simulink model "SF053A_HwAgVehCentrTrim"  (R2013b)
settings: Solver=FixedStepDiscrete  SolverMode=SingleTasking  StartTime=0.0  StopTime=1  FixedStep=0.002  RelTol=1e-3
values from neighbouring files (symbols this model uses):
  ENGRUNACTVTRUE_CNT_U08 = DataDict.Constant    [SF053A_HwAgVehCentrTrim_DataDict.m]
  HWAGCLRTRIMPRFMD_CNT_LGC = DataDict.Constant    [SF053A_HwAgVehCentrTrim_DataDict.m]
  HWAGCLRVAL_HWDEG_F32 = DataDict.Constant    [SF053A_HwAgVehCentrTrim_DataDict.m]
  HWAGEOTCCWNOTDETD_CNT_U08 = DataDict.Constant    [SF053A_HwAgVehCentrTrim_DataDict.m]
  HWAGEOTCWNOTDETD_CNT_U08 = DataDict.Constant    [SF053A_HwAgVehCentrTrim_DataDict.m]
  HWAGMAGTHDEXCDD_CNT_U08 = DataDict.Constant    [SF053A_HwAgVehCentrTrim_DataDict.m]
  HWAGTRIMPRFMD_CNT_LGC = DataDict.Constant    [SF053A_HwAgVehCentrTrim_DataDict.m]
  HwAgVehCentrTrimHwAgLim = DataDict.Calibration    [SF053A_HwAgVehCentrTrim_DataDict.m]
  HwAgVehCentrTrimVehSpdMaxThd = DataDict.Calibration    [SF053A_HwAgVehCentrTrim_DataDict.m]
  HwAgVehCentrTrimVld = DataDict.NTC    [SF053A_HwAgVehCentrTrim_DataDict.m]
  NODEBSTEP_CNT_U16 = DataDict.Constant    [SF053A_HwAgVehCentrTrim_DataDict.m]
  UPDHWAGTRIMPRFMD_CNT_U08 = DataDict.Constant    [SF053A_HwAgVehCentrTrim_DataDict.m]
  VEHSPDTHDEXCDD_CNT_U08 = DataDict.Constant    [SF053A_HwAgVehCentrTrim_DataDict.m]
undefined symbols (not defined in the file or in its folder): NtcSts1, u2, u3, u4, u5
libraries: simulink x6, NxtrNvM x3, NxtrLim x2
(part 1 of 3)
settings Model: Creator=qzwc4r  LastModifiedBy=NZ2883
settings SolverCC: AutoInsertRateTranBlk=on  InsertRTBMode=Always
settings DataIOCC: LimitDataPoints=off  SaveFormat=Structure  ReturnWorkspaceOutputs=on
settings OptimizationCC: BlockReduction=off  InlineParams=on  ZeroExternalMemoryAtStartup=off  ZeroInternalMemoryAtStartup=off  OptimizeModelRefInitCode=on  LifeSpan=1
settings DebuggingCC: SignalInfNanChecking=error  SignalRangeChecking=warning  UnderspecifiedInitializationDetection=Simplified  SolverPrmCheckMsg=error  InheritedTsInSrcMsg=error  DiscreteInheritContinuousMsg=error  SingleTaskRateTransMsg=error  TasksWithSamePriorityMsg=error  SigSpecEnsureSampleTimeMsg=error  CheckMatrixSingularityMsg=error  ParameterUnderflowMsg=error  ParameterPrecisionLossMsg=error  ParameterTunabilityLossMsg=error  FixptConstUnderflowMsg=warning  FixptConstOverflowMsg=warning  VectorMatrixConversionMsg=error  SignalLabelMismatchMsg=error  UnconnectedInputMsg=error  UnconnectedOutputMsg=error  UnconnectedLineMsg=error  SFcnCompatibilityMsg=error  UniqueDataStoreMsg=warning  BusObjectLabelMismatch=error  RootOutportRequireBusObject=error  AssertControl=DisableAll  ModelReferenceIOMsg=error  ModelReferenceVersionMismatchMessage=warning  ModelReferenceIOMismatchMessage=error  ModelReferenceCSMismatchMessage=warning  ModelReferenceDataLoggingMessage=error  StateNameClashWarn=warning  StrictBusMsg=ErrorOnBusTreatedAsVector  NonBusSignalsTreatedAsBus=error  SFUnexpectedBacktrackingDiag=error  SFInvalidInputDataAccessInChartInitDiag=error  SFNoUnconditionalDefaultTransitionDiag=error  SFTransitionOutsideNaturalParentDiag=error  SFUnconditionalTransitionShadowingDiag=error  SFUndirectedBroadcastEventsDiag=error
settings ModelReferenceCC: ModelReferenceNumInstancesAllowed=Single
settings RTWCC: SystemTargetFile=autosar.tlc  GenCodeOnly=on  TemplateMakefile=ert_default_tmf  Description=AUTOSAR  GenerateReport=on  ProcessScript=autosar_make_rtw_hook  LaunchReport=on
settings CodeAppCC: GenerateComments=off  IgnoreCustomStorageClasses=off  CustomSymbolStrType=$N$R$M  CustomSymbolStrBlkIO=$N$M  SimulinkBlockComments=off
settings STFCustomTargetCC: ParMdlRefBuildCompliant=on  CompOptLevelCompliant=on  IncludeMdlTerminateFcn=off  CombineOutputUpdateFcns=on  SuppressErrorStatus=on  ERTFirstTimeCompliant=on  ERTCustomFileBanners=on  SupportNonFinite=off  SupportComplex=off  SupportContinuousTime=off  SupportNonInlinedSFcns=off  MATLABClassNameForMDSCustomization=Simulink.SoftwareTarget.ERTCustomization  AutosarCompliant=on  GRTInterface=off  SystemTargetFile=autosar.tlc
settings ERTTargetCC: CodeReplacementLibrary=ANSI_C  ConcurrentExecutionCompliant=off  IncludeMdlTerminateFcn=off  SuppressErrorStatus=on  SupportNonFinite=off  SupportComplex=off  ModelStepFunctionPrototypeControlCompliant=off  CPPClassGenCompliant=off  AutosarCompliant=on  InlinedParameterPlacement=NonHierarchical  ERTCustomFileTemplate=example_file_process.tlc  EnableUserReplacementTypes=on

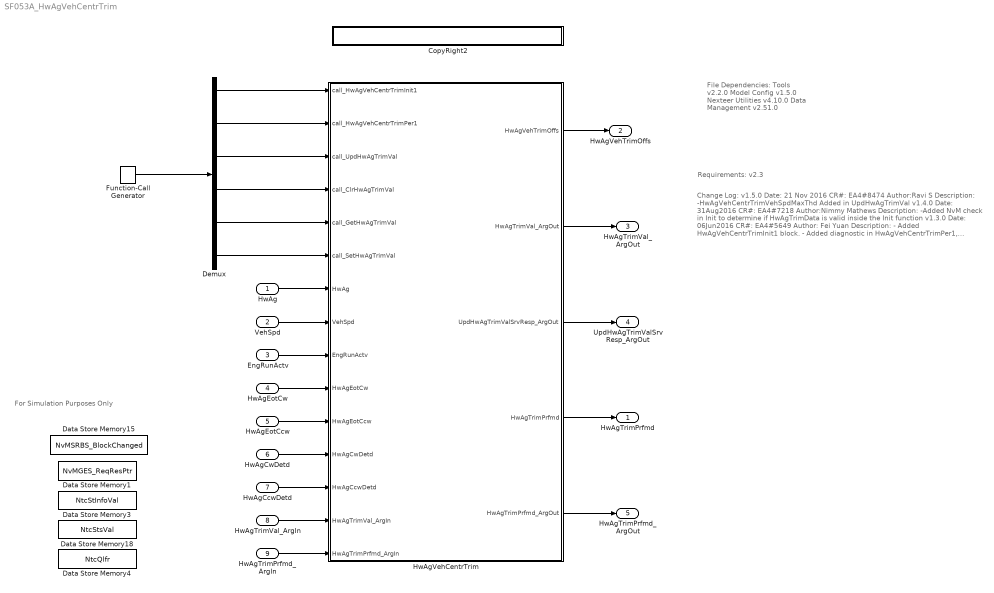
== system SF053A_HwAgVehCentrTrim ==
  note: Requirements: v2.3
  note: File Dependencies:
      | Tools v2.2.0
      | Model Config v1.5.0
      | Nexteer Utilities v4.10.0
      | Data Management v2.51.0
  note: Change Log:
      |
      | v1.5.0
      | Date: 21 Nov 2016
      | CR#: EA4#8474
      | Author:Ravi S
      | Description:
      | -HwAgVehCentrTrimVehSpdMaxThd  Added in UpdHwAgTrimVal
      |
      |
      | v1.4.0
      | Date: 31Aug2016
      | CR#: EA4#7218
      | Author:Nimmy Mathews
      | Description:
      | -Added NvM check in Init to determine if HwAgTrimData is valid inside
      | the Init function
      |
      | v1.3.0
      | Date: 06Jun2016
      | CR#: EA4#5649
      | Author: Fei Yuan
      | Description:
      | - Added HwAgVehCentrTrimInit1 block.
      | - Added diagnostic in HwAgVehCentrTrimPer1,
      |   UpdHwAgTrimVal and ClrHwAgTrimVal.
      | - Added NODEBSTEP_CNT_U16, HwAgVehCentrTrimVld
      |   HWAGVEHCENTRTRIM_HWAGVEHCENTRTRIMVLDNTCNR_CNT_ENUM.
      | - Changed the range of UpdHwAgTrimValSrvResp_ArgOut to [0,5]
      |
      | v1.2.0
      | Date: 4April2016
      | CR#: EA4#4776
      | Author: Nimmy Mathews
      | Description:
      |  - Added default value to the NVM Data Definition
      | in DD
      |
      | v1.1.0
      | Date: 30March2016
      | CR#: EA4#4776
      | Author: Nimmy Mathews
      | Description:
      |  -Added new HwAgTrimPrfmd global output and
      |  also the Trim Performed status written to NVRAM.
      | Two interface names changed
      | -HwAgEotCwDetd is renamed to HwAgCwDetd
      | -HwAgEotCcwDetd is renamed to HwAgCcwDetd
      |
      | v1.0.0
      | Date: 16Feb2016
      | CR#: EA4#3817
      | Author: Price Lefler
      | Description:
      |  - Initial Design
  note: For Simulation Purposes Only
  HwAg : Inport  RequirementInfo={} %GIDa_113f3a3e_16c4_454d_8e42_dd983b59641f
  VehSpd : Inport  RequirementInfo={} %GIDa_04c22129_0294_4664_9901_89f5670e71dd  Port=2
  EngRunActv : Inport  RequirementInfo={} %GIDa_2ca8b555_30d5_45c5_8570_785fbe8b196c  Port=3
  HwAgEotCw : Inport  RequirementInfo={} %GIDa_4439beba_6576_476c_b9c0_099ead0766d6  Port=4
  HwAgEotCcw : Inport  RequirementInfo={} %GIDa_f3262bf3_e9f3_4a2e_972e_ca5eb7281d34  Port=5
  HwAgCwDetd : Inport  RequirementInfo={} %GIDa_8f1cc708_64b7_49e1_8286_e1db8b0c7567  Port=6
  HwAgCcwDetd : Inport  RequirementInfo={} %GIDa_978389ba_efca_48a6_b124_a6774b318c9c  Port=7
  HwAgTrimVal_ArgIn : Inport  RequirementInfo={} %GIDa_c15efb6b_9d38_4c87_8d86_863040277de8  Port=8
  HwAgTrimPrfmd_ArgIn : Inport  RequirementInfo={} %GIDa_654e7d29_ce2a_48b7_b803_7a5262d5d910  Port=9
  CopyRight2 : Subsystem  Description=|  mask(Copyright Information){none=on}
      | Copyright info block.                                               
      |                                                                     
      | Place copyright information at the top of every subsystem in design.
      mask prompts: none "No parameters"
      mask help: Place copyright information at the top of every subsystem in design.
      mask Display:
      | NxtrConf = 'Nexteer Confidential';
      | 
      | sys = bdroot; %handle for the current model ("system")
      | first = get_param(sys,'Created');
      | if(isempty(first))
      |     first = datestr(now,'yyyy');
      | else
      |     first = first(end-3:end);  %year is last four digits
      | end
      | 
      | last = get_param(sys,'LastModifiedDate');
      | if isempty(last)
      |     last = datestr(now,'yyyy');
      | else
      |     last = last(end-3:end);
      | end
      | 
      | if strcmp(first,last)
      |     fprintf('%s -- Copyright %s Nexteer',NxtrConf,first)
      | else
      |     fprintf('%s -- %s%s- %s Nexteer',NxtrConf,char(169),first,last)
      | end
  Data Store Memory1 : DataStoreMemory  DataStoreName=NvMGES_ReqResPtr  OutDataTypeStr=uint8
  Data Store Memory15 : DataStoreMemory  DataStoreName=NvMSRBS_BlockChanged  VectorParams1D=off
  Data Store Memory18 : DataStoreMemory  DataStoreName=NtcStsVal  InitialValue=NtcSts1.NTCSTS_PASSD  OutDataTypeStr=Enum: NtcSts1
  Data Store Memory3 : DataStoreMemory  DataStoreName=NtcStInfoVal  OutDataTypeStr=uint8
  Data Store Memory4 : DataStoreMemory  DataStoreName=NtcQlfr  InitialValue=SigQlfr1.SIGQLFR_NORES  OutDataTypeStr=Enum: SigQlfr1
  Demux : Demux  Outputs=6
  Function-Call Generator : simulink/Ports & Subsystems/Function-Call Generator  sample_time=1  numberOfIterations=1
  HwAgVehCentrTrim : Subsystem
  HwAgTrimPrfmd : Outport
  HwAgVehTrimOffs : Outport  Port=2
  HwAgTrimVal_ArgOut : Outport  Port=3
  UpdHwAgTrimValSrvResp_ArgOut : Outport  Port=4
  HwAgTrimPrfmd_ArgOut : Outport  Port=5
  wires:
  Function-Call Generator/1 -> Demux/1
  HwAgVehCentrTrim/3(UpdHwAgTrimValSrvResp_ArgOut) -> UpdHwAgTrimValSrvResp_ArgOut/1
  HwAgVehCentrTrim/2(HwAgTrimVal_ArgOut) -> HwAgTrimVal_ArgOut/1
  HwAgVehCentrTrim/4(HwAgTrimPrfmd) -> HwAgTrimPrfmd/1
  HwAgVehCentrTrim/5(HwAgTrimPrfmd_ArgOut) -> HwAgTrimPrfmd_ArgOut/1
  Demux/3 -> HwAgVehCentrTrim/3(call_UpdHwAgTrimVal)
  Demux/4 -> HwAgVehCentrTrim/4(call_ClrHwAgTrimVal)
  Demux/2 -> HwAgVehCentrTrim/2(call_HwAgVehCentrTrimPer1)
  Demux/5 -> HwAgVehCentrTrim/5(call_GetHwAgTrimVal)
  Demux/1 -> HwAgVehCentrTrim/1(call_HwAgVehCentrTrimInit1)
  Demux/6 -> HwAgVehCentrTrim/6(call_SetHwAgTrimVal)
  HwAg/1 -> HwAgVehCentrTrim/7(HwAg)
  EngRunActv/1 -> HwAgVehCentrTrim/9(EngRunActv)
  HwAgVehCentrTrim/1(HwAgVehTrimOffs) -> HwAgVehTrimOffs/1
  VehSpd/1 -> HwAgVehCentrTrim/8(VehSpd)
  HwAgEotCw/1 -> HwAgVehCentrTrim/10(HwAgEotCw)
  HwAgEotCcw/1 -> HwAgVehCentrTrim/11(HwAgEotCcw)
  HwAgCwDetd/1 -> HwAgVehCentrTrim/12(HwAgCwDetd)
  HwAgCcwDetd/1 -> HwAgVehCentrTrim/13(HwAgCcwDetd)
  HwAgTrimVal_ArgIn/1 -> HwAgVehCentrTrim/14(HwAgTrimVal_ArgIn)
  HwAgTrimPrfmd_ArgIn/1 -> HwAgVehCentrTrim/15(HwAgTrimPrfmd_ArgIn)

== system SF053A_HwAgVehCentrTrim/CopyRight2 ==

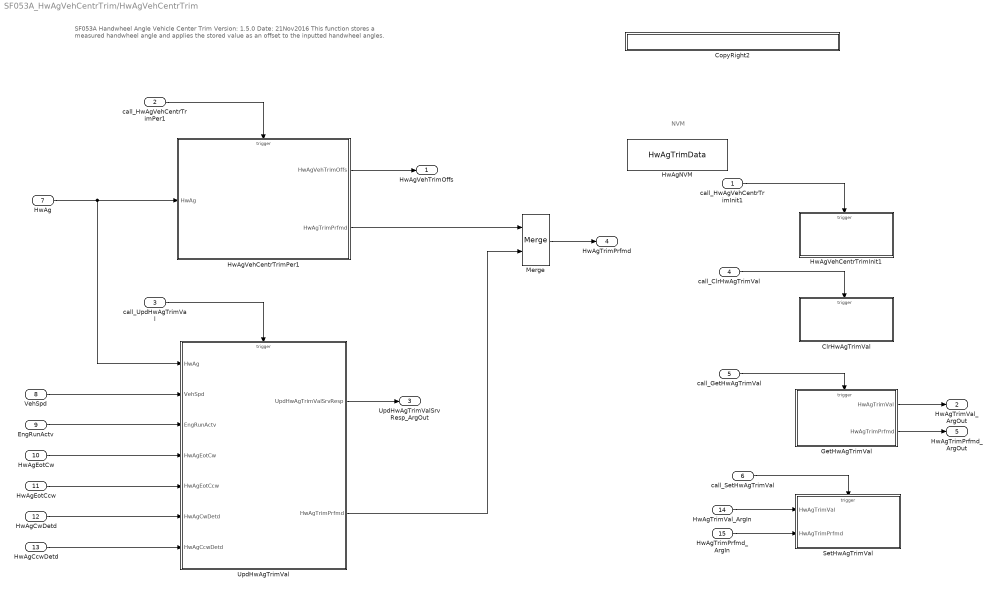
== system SF053A_HwAgVehCentrTrim/HwAgVehCentrTrim ==
  note: NVM
  note: SF053A Handwheel Angle Vehicle Center Trim
      | Version: 1.5.0	Date: 21Nov2016
      |
      | This function stores a measured handwheel angle and applies the stored value as an offset to the inputted handwheel angles.
  call_HwAgVehCentrTrimInit1 : Inport  RequirementInfo="{'linktype_rmi_doors' '0000babb (/E-STEER Core/SubSystem Specifications/Application Functions/SF053A Handwheel Angle Vehicle Center Trim)' '#SF053A_64' 'true' 'REQ:  SF053A_64' '' } %GIDa_f9a0f12b_42b7_4d6c_834e_7e4278808bcd"
  call_HwAgVehCentrTrimPer1 : Inport  RequirementInfo="{'linktype_rmi_doors' '0000babb (/E-STEER Core/SubSystem Specifications/Application Functions/SF053A Handwheel Angle Vehicle Center Trim)' '#SF053A_53' 'true' 'REQ:  SF053A_53' '' } %GIDa_b7a3059f_f6a3_46c4_b182_932d9e52892f"  Port=2
  call_UpdHwAgTrimVal : Inport  RequirementInfo="{'linktype_rmi_doors' '0000babb (/E-STEER Core/SubSystem Specifications/Application Functions/SF053A Handwheel Angle Vehicle Center Trim)' '#SF053A_79' 'true' 'REQ:  SF053A_79' '' } %GIDa_62e46fcf_ea6a_4b4f_93c9_5136d417b28b"  Port=3
  call_ClrHwAgTrimVal : Inport  RequirementInfo="{'linktype_rmi_doors' '0000babb (/E-STEER Core/SubSystem Specifications/Application Functions/SF053A Handwheel Angle Vehicle Center Trim)' '#SF053A_64' 'true' 'REQ:  SF053A_64' '' } %GIDa_a2a55ca3_d233_4c8c_83e4_64e16e91eece"  Port=4
  call_GetHwAgTrimVal : Inport  RequirementInfo="{'linktype_rmi_doors' '0000babb (/E-STEER Core/SubSystem Specifications/Application Functions/SF053A Handwheel Angle Vehicle Center Trim)' '#SF053A_62' 'true' 'REQ:  SF053A_62' '' } %GIDa_c620757b_2c38_453b_8133_45c36bdcdd0e"  Port=5
  call_SetHwAgTrimVal : Inport  RequirementInfo="{'linktype_rmi_doors' '0000babb (/E-STEER Core/SubSystem Specifications/Application Functions/SF053A Handwheel Angle Vehicle Center Trim)' '#SF053A_59' 'true' 'REQ:  SF053A_59' '' } %GIDa_33d0015f_790b_4486_865d_38381a9ea06a"  Port=6
  HwAg : Inport  RequirementInfo="{'linktype_rmi_doors' '0000babb (/E-STEER Core/SubSystem Specifications/Application Functions/SF053A Handwheel Angle Vehicle Center Trim)' '#SF053A_10' 'true' 'REQ:  SF053A_10' '' } %GIDa_b0128c29_6a82_43ee_9dda_c0c68b77b530"  Port=7
  VehSpd : Inport  RequirementInfo="{'linktype_rmi_doors' '0000babb (/E-STEER Core/SubSystem Specifications/Application Functions/SF053A Handwheel Angle Vehicle Center Trim)' '#SF053A_11' 'true' 'REQ:  SF053A_11' '' } %GIDa_a57cdbec_173c_4b3b_a957_fb6f740bfc19"  Port=8
  EngRunActv : Inport  RequirementInfo="{'linktype_rmi_doors' '0000babb (/E-STEER Core/SubSystem Specifications/Application Functions/SF053A Handwheel Angle Vehicle Center Trim)' '#SF053A_12' 'true' 'REQ:  SF053A_12' '' } %GIDa_2bbfd2af_ef79_4ac0_8512_672b914117e8"  Port=9
  HwAgEotCw : Inport  RequirementInfo="{'linktype_rmi_doors' '0000babb (/E-STEER Core/SubSystem Specifications/Application Functions/SF053A Handwheel Angle Vehicle Center Trim)' '#SF053A_13' 'true' 'REQ:  SF053A_13' '' } %GIDa_f43d4b7f_acdd_4c76_aa56_82bfdd82067a"  Port=10
  HwAgEotCcw : Inport  RequirementInfo="{'linktype_rmi_doors' '0000babb (/E-STEER Core/SubSystem Specifications/Application Functions/SF053A Handwheel Angle Vehicle Center Trim)' '#SF053A_14' 'true' 'REQ:  SF053A_14' '' } %GIDa_e1dc5bbe_2182_488e_9f21_c5e98eb0726c"  Port=11
  HwAgCwDetd : Inport  RequirementInfo="{'linktype_rmi_doors' '0000babb (/E-STEER Core/SubSystem Specifications/Application Functions/SF053A Handwheel Angle Vehicle Center Trim)' '#SF053A_15' 'true' 'REQ:  SF053A_15' '' } %GIDa_9b93c2bf_36b3_43d6_8875_515dee61e84b"  Port=12
  HwAgCcwDetd : Inport  RequirementInfo="{'linktype_rmi_doors' '0000babb (/E-STEER Core/SubSystem Specifications/Application Functions/SF053A Handwheel Angle Vehicle Center Trim)' '#SF053A_16' 'true' 'REQ:  SF053A_16' '' } %GIDa_d87faf20_2cd4_4771_90c3_b7a20e388060"  Port=13
  HwAgTrimVal_ArgIn : Inport  RequirementInfo="{'linktype_rmi_doors' '0000babb (/E-STEER Core/SubSystem Specifications/Application Functions/SF053A Handwheel Angle Vehicle Center Trim)' '#SF053A_59' 'true' 'REQ:  SF053A_59' '' } %GIDa_aee0353a_4813_42ed_8b25_32aaed297abf"  Port=14
  HwAgTrimPrfmd_ArgIn : Inport  RequirementInfo="{'linktype_rmi_doors' '0000babb (/E-STEER Core/SubSystem Specifications/Application Functions/SF053A Handwheel Angle Vehicle Center Trim)' '#SF053A_59' 'true' 'REQ:  SF053A_59' '' } %GIDa_1c050af2_beaf_4e57_9801_0facf100b431"  Port=15
  ClrHwAgTrimVal : Subsystem  RequirementInfo="{'linktype_rmi_doors' '0000babb (/E-STEER Core/SubSystem Specifications/Application Functions/SF053A Handwheel Angle Vehicle Center Trim)' '#SF053A_64' 'true' 'REQ:  SF053A_64' '' } %GIDa_29cbfc29_7db8_4849_9914_e3195bd45596"  TreatAsAtomicUnit=on
  CopyRight2 : Subsystem  Description=|  mask(Copyright Information){none=on}
      | Copyright info block.                                               
      |                                                                     
      | Place copyright information at the top of every subsystem in design.
      mask prompts: none "No parameters"
      mask help: Place copyright information at the top of every subsystem in design.
      mask Display:
      | NxtrConf = 'Nexteer Confidential';
      | 
      | sys = bdroot; %handle for the current model ("system")
      | first = get_param(sys,'Created');
      | if(isempty(first))
      |     first = datestr(now,'yyyy');
      | else
      |     first = first(end-3:end);  %year is last four digits
      | end
      | 
      | last = get_param(sys,'LastModifiedDate');
      | if isempty(last)
      |     last = datestr(now,'yyyy');
      | else
      |     last = last(end-3:end);
      | end
      | 
      | if strcmp(first,last)
      |     fprintf('%s -- Copyright %s Nexteer',NxtrConf,first)
      | else
      |     fprintf('%s -- %s%s- %s Nexteer',NxtrConf,char(169),first,last)
      | end
  GetHwAgTrimVal : Subsystem  RequirementInfo="{'linktype_rmi_doors' '0000babb (/E-STEER Core/SubSystem Specifications/Application Functions/SF053A Handwheel Angle Vehicle Center Trim)' '#SF053A_62' 'true' 'REQ:  SF053A_62' '' } %GIDa_76c2d87e_e8ee_4f7f_ac2c_f7e43012ac53"  TreatAsAtomicUnit=on
  HwAgNVM : DataStoreMemory  DataStoreName=HwAgTrimData  InitialValue=[]  OutDataTypeStr=Bus: HwAgSnsrTrimRec1  StateMustResolveToSignalObject=on
  HwAgVehCentrTrimInit1 : Subsystem  RequirementInfo="{'linktype_rmi_doors' '0000babb (/E-STEER Core/SubSystem Specifications/Application Functions/SF053A Handwheel Angle Vehicle Center Trim)' '#SF053A_55' 'true' 'REQ:  SF053A_55' '' } %GIDa_87096361_849b_43ed_ad0b_91d28511535a"  TreatAsAtomicUnit=on
  HwAgVehCentrTrimPer1 : Subsystem  TreatAsAtomicUnit=on
  Merge : Merge  RequirementInfo="{'linktype_rmi_doors' '0000babb (/E-STEER Core/SubSystem Specifications/Application Functions/SF053A Handwheel Angle Vehicle Center Trim)' '#SF053A_86' 'true' 'REQ:  SF053A_86' '' } %GIDa_bbe5d05c_97ec_4738_8cf7_2eeb84dd25f0"
  SetHwAgTrimVal : Subsystem  RequirementInfo="{'linktype_rmi_doors' '0000babb (/E-STEER Core/SubSystem Specifications/Application Functions/SF053A Handwheel Angle Vehicle Center Trim)' '#SF053A_59' 'true' 'REQ:  SF053A_59' '' } %GIDa_073a05b8_7576_4716_bba7_b0a32cf448e1"  TreatAsAtomicUnit=on
  UpdHwAgTrimVal : Subsystem  RequirementInfo="{'linktype_rmi_doors' '0000babb (/E-STEER Core/SubSystem Specifications/Application Functions/SF053A Handwheel Angle Vehicle Center Trim)' '#SF053A_67' 'true' 'REQ:  SF053A_67' '' ; 'linktype_rmi_doors' '0000babb (/E-STEER Core/SubSystem Specifications/Application Functions/SF053A Handwheel Angle Vehicle Center Trim)' '#SF053A_33' 'true' 'REQ:  SF053A_33' '' } %GIDa_c063e4fc_1dad_4a60_a62c_b14edd11c2e7"  TreatAsAtomicUnit=on
  HwAgVehTrimOffs : Outport  RequirementInfo="{'linktype_rmi_doors' '0000babb (/E-STEER Core/SubSystem Specifications/Application Functions/SF053A Handwheel Angle Vehicle Center Trim)' '#SF053A_19' 'true' 'REQ:  SF053A_19' '' ; 'linktype_rmi_doors' '0000babb (/E-STEER Core/SubSystem Specifications/Application Functions/SF053A Handwheel Angle Vehicle Center Trim)' '#SF053A_65' 'true' 'REQ:  SF053A_65' '' ; 'linktype_rmi_doors' '0000babb (/E-STEER Core/SubSystem Specifications/Application Functions/SF053A Handwheel Angle Vehicle Center Trim)' '#SF053A_47' 'true' 'REQ:  SF053A_47' '' } %GIDa_dcfa4732_c568_4e6d_aa39_ecb4cb0257dc"
  HwAgTrimVal_ArgOut : Outport  RequirementInfo="{'linktype_rmi_doors' '0000babb (/E-STEER Core/SubSystem Specifications/Application Functions/SF053A Handwheel Angle Vehicle Center Trim)' '#SF053A_62' 'true' 'REQ:  SF053A_62' '' } %GIDa_05d1222d_295a_473c_9d17_a3b3cf33a958"  Port=2
  UpdHwAgTrimValSrvResp_ArgOut : Outport  Port=3
  HwAgTrimPrfmd : Outport  RequirementInfo="{'linktype_rmi_doors' '0000babb (/E-STEER Core/SubSystem Specifications/Application Functions/SF053A Handwheel Angle Vehicle Center Trim)' '#SF053A_86' 'true' 'REQ:  SF053A_86' '' ; 'linktype_rmi_doors' '0000babb (/E-STEER Core/SubSystem Specifications/Application Functions/SF053A Handwheel Angle Vehicle Center Trim)' '#SF053A_90' 'true' 'REQ:  SF053A_90' '' } %GIDa_ea1254c4_d164_44f0_a5de_e3baab78e443"  Port=4
  HwAgTrimPrfmd_ArgOut : Outport  RequirementInfo="{'linktype_rmi_doors' '0000babb (/E-STEER Core/SubSystem Specifications/Application Functions/SF053A Handwheel Angle Vehicle Center Trim)' '#SF053A_62' 'true' 'REQ:  SF053A_62' '' } %GIDa_06da9a76_07ff_4c32_a1be_6e57f94593db"  Port=5
  wires:
  HwAg/1 -> UpdHwAgTrimVal/1(HwAg), HwAgVehCentrTrimPer1/1(HwAg)
  VehSpd/1 -> UpdHwAgTrimVal/2(VehSpd)
  EngRunActv/1 -> UpdHwAgTrimVal/3(EngRunActv)
  HwAgEotCw/1 -> UpdHwAgTrimVal/4(HwAgEotCw)
  HwAgEotCcw/1 -> UpdHwAgTrimVal/5(HwAgEotCcw)
  HwAgCwDetd/1 -> UpdHwAgTrimVal/6(HwAgCwDetd)
  HwAgCcwDetd/1 -> UpdHwAgTrimVal/7(HwAgCcwDetd)
  call_HwAgVehCentrTrimPer1/1 -> HwAgVehCentrTrimPer1/Trigger
  call_UpdHwAgTrimVal/1 -> UpdHwAgTrimVal/Trigger
  HwAgTrimVal_ArgIn/1 -> SetHwAgTrimVal/1(HwAgTrimVal)
  GetHwAgTrimVal/1(HwAgTrimVal) -> HwAgTrimVal_ArgOut/1
  UpdHwAgTrimVal/1(UpdHwAgTrimValSrvResp) -> UpdHwAgTrimValSrvResp_ArgOut/1
  HwAgVehCentrTrimPer1/1(HwAgVehTrimOffs) -> HwAgVehTrimOffs/1
  call_ClrHwAgTrimVal/1 -> ClrHwAgTrimVal/Trigger
  call_GetHwAgTrimVal/1 -> GetHwAgTrimVal/Trigger
  call_SetHwAgTrimVal/1 -> SetHwAgTrimVal/Trigger
  UpdHwAgTrimVal/2(HwAgTrimPrfmd) -> Merge/2
  Merge/1 -> HwAgTrimPrfmd/1
  HwAgVehCentrTrimPer1/2(HwAgTrimPrfmd) -> Merge/1
  GetHwAgTrimVal/2(HwAgTrimPrfmd) -> HwAgTrimPrfmd_ArgOut/1
  HwAgTrimPrfmd_ArgIn/1 -> SetHwAgTrimVal/2(HwAgTrimPrfmd)
  call_HwAgVehCentrTrimInit1/1 -> HwAgVehCentrTrimInit1/Trigger

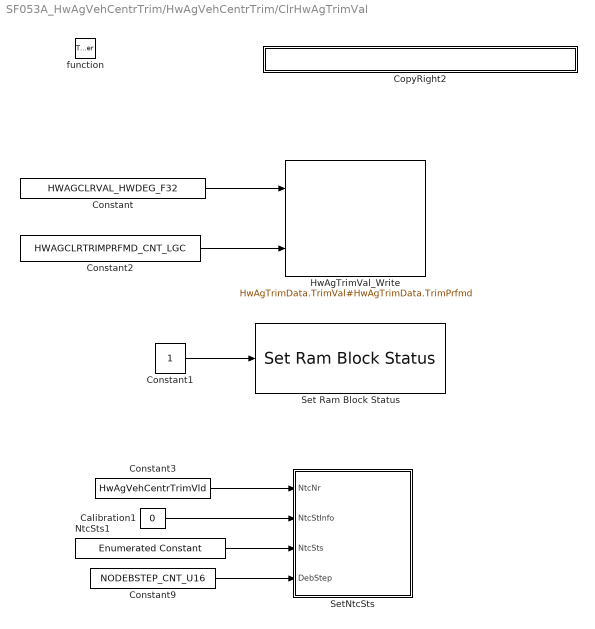
== system SF053A_HwAgVehCentrTrim/HwAgVehCentrTrim/ClrHwAgTrimVal ==
  function : TriggerPort  TriggerType=function-call
  Calibration1 : Constant  RequirementInfo="{'linktype_rmi_doors' '0000babb (/E-STEER Core/SubSystem Specifications/Application Functions/SF053A Handwheel Angle Vehicle Center Trim)' '#SF053A_114' 'true' 'REQ:  SF053A_114' '' } %GIDa_e2bf0df4_8061_4554_9723_0bf4b0608522"  Value=0  OutDataTypeStr=uint8
      settings: AttributesFormatString=%<OutDataTypeStr>
  Constant : Constant  RequirementInfo="{'linktype_rmi_doors' '0000babb (/E-STEER Core/SubSystem Specifications/Application Functions/SF053A Handwheel Angle Vehicle Center Trim)' '#SF053A_64' 'true' 'REQ:  SF053A_64' '' } %GIDa_99bb31d9_7332_4c2b_910a_7d292128470c"  Value=HWAGCLRVAL_HWDEG_F32
  Constant1 : Constant  RequirementInfo="{'linktype_rmi_doors' '0000babb (/E-STEER Core/SubSystem Specifications/Application Functions/SF053A Handwheel Angle Vehicle Center Trim)' '#SF053A_92' 'true' 'REQ:  SF053A_92' '' } %GIDa_021d6c99_15c2_441d_bed0_39bcbafdbdbf"  OutDataTypeStr=uint8
  Constant2 : Constant  RequirementInfo="{'linktype_rmi_doors' '0000babb (/E-STEER Core/SubSystem Specifications/Application Functions/SF053A Handwheel Angle Vehicle Center Trim)' '#SF053A_92' 'true' 'REQ:  SF053A_92' '' ; 'linktype_rmi_doors' '0000babb (/E-STEER Core/SubSystem Specifications/Application Functions/SF053A Handwheel Angle Vehicle Center Trim)' '#SF053A_8' 'true' 'REQ:  SF053A_8' '' } %GIDa_d79a27e5_3809_434e_a549_54ecca6b715b"  Value=HWAGCLRTRIMPRFMD_CNT_LGC
  Constant3 : Constant  RequirementInfo="{'linktype_rmi_doors' '0000babb (/E-STEER Core/SubSystem Specifications/Application Functions/SF053A Handwheel Angle Vehicle Center Trim)' '#SF053A_92' 'true' 'REQ:  SF053A_92' '' ; 'linktype_rmi_doors' '0000babb (/E-STEER Core/SubSystem Specifications/Application Functions/SF053A Handwheel Angle Vehicle Center Trim)' '#SF053A_114' 'true' 'REQ:  SF053A_114' '' } %GIDa_6e6052d3_f7df_4117_b214_7e6538016c26"  Value=HwAgVehCentrTrimVld
  Constant9 : Constant  RequirementInfo="{'linktype_rmi_doors' '0000babb (/E-STEER Core/SubSystem Specifications/Application Functions/SF053A Handwheel Angle Vehicle Center Trim)' '#SF053A_114' 'true' 'REQ:  SF053A_114' '' } %GIDa_b5a8c722_2206_4b38_b068_a44dc0b84817"  Value=NODEBSTEP_CNT_U16
  CopyRight2 : Subsystem  Description=|  mask(Copyright Information){none=on}
      | Copyright info block.                                               
      |                                                                     
      | Place copyright information at the top of every subsystem in design.
      mask prompts: none "No parameters"
      mask help: Place copyright information at the top of every subsystem in design.
      mask Display:
      | NxtrConf = 'Nexteer Confidential';
      | 
      | sys = bdroot; %handle for the current model ("system")
      | first = get_param(sys,'Created');
      | if(isempty(first))
      |     first = datestr(now,'yyyy');
      | else
      |     first = first(end-3:end);  %year is last four digits
      | end
      | 
      | last = get_param(sys,'LastModifiedDate');
      | if isempty(last)
      |     last = datestr(now,'yyyy');
      | else
      |     last = last(end-3:end);
      | end
      | 
      | if strcmp(first,last)
      |     fprintf('%s -- Copyright %s Nexteer',NxtrConf,first)
      | else
      |     fprintf('%s -- %s%s- %s Nexteer',NxtrConf,char(169),first,last)
      | end
  HwAgTrimVal_Write : DataStoreWrite  RequirementInfo="{'linktype_rmi_doors' '0000babb (/E-STEER Core/SubSystem Specifications/Application Functions/SF053A Handwheel Angle Vehicle Center Trim)' '#SF053A_92' 'true' 'REQ:  SF053A_92' '' ; 'linktype_rmi_doors' '0000babb (/E-STEER Core/SubSystem Specifications/Application Functions/SF053A Handwheel Angle Vehicle Center Trim)' '#SF053A_64' 'true' 'REQ:  SF053A_64' '' ; 'linktype_rmi_doors' '0000babb (/E-STEER Core/SubSystem Specifications/Application Functions/SF053A Handwheel Angle Vehicle Center Trim)' '#SF053A_8' 'true' 'REQ:  SF053A_8' '' } %GIDa_2ae5e603_6939_4147_8c91_2053cf458421"  DataStoreName=HwAgTrimData  DataStoreElements=HwAgTrimData.TrimVal#HwAgTrimData.TrimPrfmd
  NtcSts1 : simulink/Sources/Enumerated Constant  RequirementInfo="{'linktype_rmi_doors' '0000babb (/E-STEER Core/SubSystem Specifications/Application Functions/SF053A Handwheel Angle Vehicle Center Trim)' '#SF053A_114' 'true' 'REQ:  SF053A_114' '' } %GIDa_6f141e7f_1637_49b4_932f_33a27434162f"  OutDataTypeStr=Enum: NtcSts1  Value=NtcSts1.NTCSTS_FAILD  SampleTime=inf
  Set Ram Block Status : NxtrNvM/Set Ram Block Status  RequirementInfo="{'linktype_rmi_doors' '0000babb (/E-STEER Core/SubSystem Specifications/Application Functions/SF053A Handwheel Angle Vehicle Center Trim)' '#SF053A_92' 'true' 'REQ:  SF053A_92' '' } %GIDa_65d25fa0_48e8_4dea_8981_e2d0a09d197e"  FuncName=Set Ram Block Status  NvMBlockName=HwAgTrimData  VoidFuncRtn=on  BlockChanged_DSN=NvMSRBS_BlockChanged  Return_DSN=NvMSRBS_Return
      settings: AttributesFormatString=%<FuncName>
  SetNtcSts : Subsystem  RequirementInfo="{'linktype_rmi_doors' '0000babb (/E-STEER Core/SubSystem Specifications/Application Functions/SF053A Handwheel Angle Vehicle Center Trim)' '#SF053A_114' 'true' 'REQ:  SF053A_114' '' } %GIDa_8a2b31b3_439d_490b_95d1_1edec1630dcd"  TreatAsAtomicUnit=on  mask(SetNTC){}
      mask help: SetNTC library block
      settings: RTWSystemCode=Inline
  wires:
  Constant3/1 -> SetNtcSts/1(NtcNr)
  Constant/1 -> HwAgTrimVal_Write/1
  Constant1/1 -> Set Ram Block Status/1
  Constant2/1 -> HwAgTrimVal_Write/2
  NtcSts1/1 -> SetNtcSts/3(NtcSts)
  Constant9/1 -> SetNtcSts/4(DebStep)
  Calibration1/1 -> SetNtcSts/2(NtcStInfo)

== system SF053A_HwAgVehCentrTrim/HwAgVehCentrTrim/CopyRight2 ==

== system SF053A_HwAgVehCentrTrim/HwAgVehCentrTrim/GetHwAgTrimVal ==
  function : TriggerPort  TriggerType=function-call
  CopyRight2 : Subsystem  Description=|  mask(Copyright Information){none=on}
      | Copyright info block.                                               
      |                                                                     
      | Place copyright information at the top of every subsystem in design.
      mask prompts: none "No parameters"
      mask help: Place copyright information at the top of every subsystem in design.
      mask Display:
      | NxtrConf = 'Nexteer Confidential';
      | 
      | sys = bdroot; %handle for the current model ("system")
      | first = get_param(sys,'Created');
      | if(isempty(first))
      |     first = datestr(now,'yyyy');
      | else
      |     first = first(end-3:end);  %year is last four digits
      | end
      | 
      | last = get_param(sys,'LastModifiedDate');
      | if isempty(last)
      |     last = datestr(now,'yyyy');
      | else
      |     last = last(end-3:end);
      | end
      | 
      | if strcmp(first,last)
      |     fprintf('%s -- Copyright %s Nexteer',NxtrConf,first)
      | else
      |     fprintf('%s -- %s%s- %s Nexteer',NxtrConf,char(169),first,last)
      | end
  HwAgTrimData_Read : DataStoreRead  RequirementInfo="{'linktype_rmi_doors' '0000babb (/E-STEER Core/SubSystem Specifications/Application Functions/SF053A Handwheel Angle Vehicle Center Trim)' '#SF053A_62' 'true' 'REQ:  SF053A_62' '' } %GIDa_810bd88d_a327_4af3_9508_737ea4036050"  DataStoreName=HwAgTrimData  DataStoreElements=HwAgTrimData.TrimVal#HwAgTrimData.TrimPrfmd
  HwAgTrimVal : Outport  RequirementInfo="{'linktype_rmi_doors' '0000babb (/E-STEER Core/SubSystem Specifications/Application Functions/SF053A Handwheel Angle Vehicle Center Trim)' '#SF053A_62' 'true' 'REQ:  SF053A_62' '' } %GIDa_26482804_e9d8_4a70_8063_7bf3a9b37d28"
  HwAgTrimPrfmd : Outport  RequirementInfo="{'linktype_rmi_doors' '0000babb (/E-STEER Core/SubSystem Specifications/Application Functions/SF053A Handwheel Angle Vehicle Center Trim)' '#SF053A_94' 'true' 'REQ:  SF053A_94' '' } %GIDa_19e959e4_7336_4de0_a86b_6b855d337748"  Port=2
  wires:
  HwAgTrimData_Read/1 -> HwAgTrimVal/1
  HwAgTrimData_Read/2 -> HwAgTrimPrfmd/1

== system SF053A_HwAgVehCentrTrim/HwAgVehCentrTrim/HwAgVehCentrTrimInit1 ==
  function : TriggerPort  TriggerType=function-call
  Calibration1 : Constant  RequirementInfo="{'linktype_rmi_doors' '0000babb (/E-STEER Core/SubSystem Specifications/Application Functions/SF053A Handwheel Angle Vehicle Center Trim)' '#SF053A_111' 'true' 'REQ:  SF053A_111' '' } %GIDa_0ce2f3ca_f5f7_4cab_8005_506b2343ec04"  Value=0  OutDataTypeStr=uint8
      settings: AttributesFormatString=%<OutDataTypeStr>
  Constant3 : Constant  RequirementInfo="{'linktype_rmi_doors' '0000babb (/E-STEER Core/SubSystem Specifications/Application Functions/SF053A Handwheel Angle Vehicle Center Trim)' '#SF053A_111' 'true' 'REQ:  SF053A_111' '' } %GIDa_7c575ac1_99f8_41b7_bb1a_af84279c8eb5"  Value=HwAgVehCentrTrimVld
  Constant9 : Constant  RequirementInfo="{'linktype_rmi_doors' '0000babb (/E-STEER Core/SubSystem Specifications/Application Functions/SF053A Handwheel Angle Vehicle Center Trim)' '#SF053A_111' 'true' 'REQ:  SF053A_111' '' } %GIDa_3e864ee3_3992_4820_b875_987b5510025d"  Value=NODEBSTEP_CNT_U16
  CopyRight2 : Subsystem  Description=|  mask(Copyright Information){none=on}
      | Copyright info block.                                               
      |                                                                     
      | Place copyright information at the top of every subsystem in design.
      mask prompts: none "No parameters"
      mask help: Place copyright information at the top of every subsystem in design.
      mask Display:
      | NxtrConf = 'Nexteer Confidential';
      | 
      | sys = bdroot; %handle for the current model ("system")
      | first = get_param(sys,'Created');
      | if(isempty(first))
      |     first = datestr(now,'yyyy');
      | else
      |     first = first(end-3:end);  %year is last four digits
      | end
      | 
      | last = get_param(sys,'LastModifiedDate');
      | if isempty(last)
      |     last = datestr(now,'yyyy');
      | else
      |     last = last(end-3:end);
      | end
      | 
      | if strcmp(first,last)
      |     fprintf('%s -- Copyright %s Nexteer',NxtrConf,first)
      | else
      |     fprintf('%s -- %s%s- %s Nexteer',NxtrConf,char(169),first,last)
      | end
  HwAgTrimData_Read : DataStoreRead  RequirementInfo="{'linktype_rmi_doors' '0000babb (/E-STEER Core/SubSystem Specifications/Application Functions/SF053A Handwheel Angle Vehicle Center Trim)' '#SF053A_111' 'true' 'REQ:  SF053A_111' '' } %GIDa_9c2f8d01_eac2_4d00_a580_88c0c36f4950"  DataStoreName=HwAgTrimData  DataStoreElements=HwAgTrimData.TrimPrfmd
  If : If  RequirementInfo="{'linktype_rmi_doors' '0000babb (/E-STEER Core/SubSystem Specifications/Application Functions/SF053A Handwheel Angle Vehicle Center Trim)' '#SF053A_111' 'true' 'REQ:  SF053A_111' '' } %GIDa_87553632_729e_49a3_99cf_3b8744247b6e"  IfExpression=u1  ShowElse=off
  NtcSts1 : simulink/Sources/Enumerated Constant  RequirementInfo="{'linktype_rmi_doors' '0000babb (/E-STEER Core/SubSystem Specifications/Application Functions/SF053A Handwheel Angle Vehicle Center Trim)' '#SF053A_111' 'true' 'REQ:  SF053A_111' '' } %GIDa_a792af0b_da38_4a2e_87c1_7d1fd06d2788"  OutDataTypeStr=Enum: NtcSts1  Value=NtcSts1.NTCSTS_PASSD  SampleTime=inf
  SetNtcSts : Subsystem  RequirementInfo="{'linktype_rmi_doors' '0000babb (/E-STEER Core/SubSystem Specifications/Application Functions/SF053A Handwheel Angle Vehicle Center Trim)' '#SF053A_111' 'true' 'REQ:  SF053A_111' '' } %GIDa_4e333d1b_448e_4296_9aaf_a06eb46d2c97"  mask(SetNTC){}
      mask help: SetNTC library block
  wires:
  HwAgTrimData_Read/1 -> If/1
  Constant3/1 -> SetNtcSts/1(NtcNr)
  NtcSts1/1 -> SetNtcSts/3(NtcSts)
  Constant9/1 -> SetNtcSts/4(DebStep)
  Calibration1/1 -> SetNtcSts/2(NtcStInfo)
  If/1 -> SetNtcSts/Action

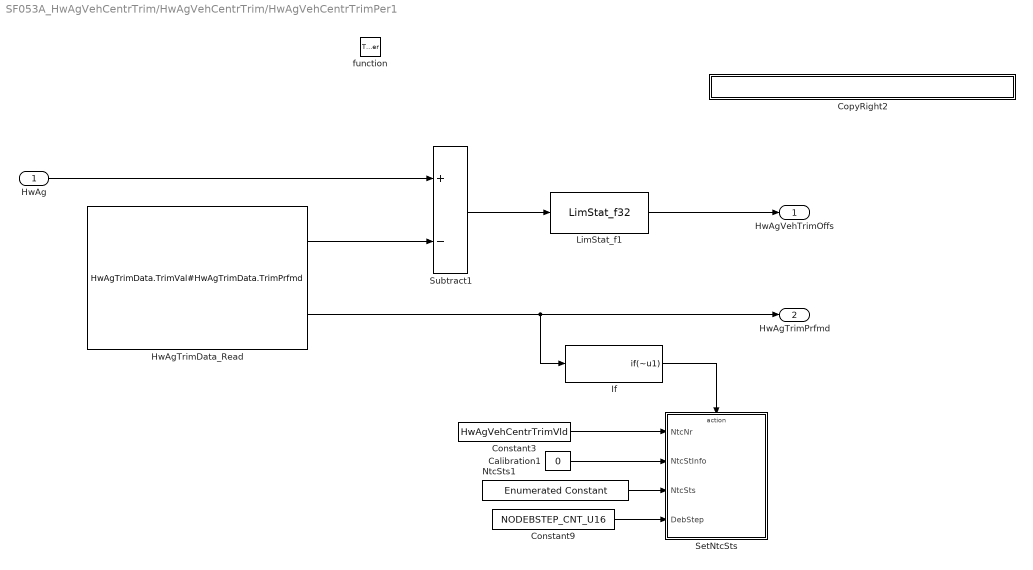
== system SF053A_HwAgVehCentrTrim/HwAgVehCentrTrim/HwAgVehCentrTrimPer1 ==
  HwAg : Inport  RequirementInfo="{'linktype_rmi_doors' '0000babb (/E-STEER Core/SubSystem Specifications/Application Functions/SF053A Handwheel Angle Vehicle Center Trim)' '#SF053A_28' 'true' 'REQ:  SF053A_28' '' } %GIDa_2271ee09_f6a8_4abb_984d_d435c9e94e26"
  function : TriggerPort  TriggerType=function-call
  Calibration1 : Constant  RequirementInfo="{'linktype_rmi_doors' '0000babb (/E-STEER Core/SubSystem Specifications/Application Functions/SF053A Handwheel Angle Vehicle Center Trim)' '#SF053A_114' 'true' 'REQ:  SF053A_114' '' } %GIDa_571dc270_8baa_4a0f_bb29_dc087c5b0725"  Value=0  OutDataTypeStr=uint8
      settings: AttributesFormatString=%<OutDataTypeStr>
  Constant3 : Constant  RequirementInfo="{'linktype_rmi_doors' '0000babb (/E-STEER Core/SubSystem Specifications/Application Functions/SF053A Handwheel Angle Vehicle Center Trim)' '#SF053A_114' 'true' 'REQ:  SF053A_114' '' } %GIDa_764e7a65_3444_4588_98a2_72e7c999fec1"  Value=HwAgVehCentrTrimVld
  Constant9 : Constant  RequirementInfo="{'linktype_rmi_doors' '0000babb (/E-STEER Core/SubSystem Specifications/Application Functions/SF053A Handwheel Angle Vehicle Center Trim)' '#SF053A_114' 'true' 'REQ:  SF053A_114' '' } %GIDa_572635a1_a779_4686_b511_91770c1f8509"  Value=NODEBSTEP_CNT_U16
  CopyRight2 : Subsystem  Description=|  mask(Copyright Information){none=on}
      | Copyright info block.                                               
      |                                                                     
      | Place copyright information at the top of every subsystem in design.
      mask prompts: none "No parameters"
      mask help: Place copyright information at the top of every subsystem in design.
      mask Display:
      | NxtrConf = 'Nexteer Confidential';
      | 
      | sys = bdroot; %handle for the current model ("system")
      | first = get_param(sys,'Created');
      | if(isempty(first))
      |     first = datestr(now,'yyyy');
      | else
      |     first = first(end-3:end);  %year is last four digits
      | end
      | 
      | last = get_param(sys,'LastModifiedDate');
      | if isempty(last)
      |     last = datestr(now,'yyyy');
      | else
      |     last = last(end-3:end);
      | end
      | 
      | if strcmp(first,last)
      |     fprintf('%s -- Copyright %s Nexteer',NxtrConf,first)
      | else
      |     fprintf('%s -- %s%s- %s Nexteer',NxtrConf,char(169),first,last)
      | end
  HwAgTrimData_Read : DataStoreRead  RequirementInfo="{'linktype_rmi_doors' '0000babb (/E-STEER Core/SubSystem Specifications/Application Functions/SF053A Handwheel Angle Vehicle Center Trim)' '#SF053A_28' 'true' 'REQ:  SF053A_28' '' } %GIDa_e3a3af1d_b7ae_447f_9fa4_0bf015972bf9"  DataStoreName=HwAgTrimData  DataStoreElements=HwAgTrimData.TrimVal#HwAgTrimData.TrimPrfmd
  If : If  RequirementInfo="{'linktype_rmi_doors' '0000babb (/E-STEER Core/SubSystem Specifications/Application Functions/SF053A Handwheel Angle Vehicle Center Trim)' '#SF053A_114' 'true' 'REQ:  SF053A_114' '' } %GIDa_035d0236_b98d_464f_b766_fd4def8204b9"  IfExpression=~u1  ShowElse=off
  LimStat_f1 : NxtrLim/LimStat_f32  Tag=Lim_f32  RequirementInfo="{'linktype_rmi_doors' '0000babb (/E-STEER Core/SubSystem Specifications/Application Functions/SF053A Handwheel Angle Vehicle Center Trim)' '#SF053A_28' 'true' 'REQ:  SF053A_28' '' } %GIDa_f6e845cc_f7fd_4300_80e1_2e360d821c59"  LoLim=SYSGLBPRM_HWAGLOLIM_HWDEG_F32  HiLim=SYSGLBPRM_HWAGHILIM_HWDEG_F32
      settings: AttributesFormatString=|
      | %<Tag>
      | Low Limit: %<LoLim>
      | High Limit:%<HiLim>
  NtcSts1 : simulink/Sources/Enumerated Constant  RequirementInfo="{'linktype_rmi_doors' '0000babb (/E-STEER Core/SubSystem Specifications/Application Functions/SF053A Handwheel Angle Vehicle Center Trim)' '#SF053A_114' 'true' 'REQ:  SF053A_114' '' } %GIDa_2897d868_a6b8_419b_b0bc_cc8cdb8f8bdc"  OutDataTypeStr=Enum: NtcSts1  Value=NtcSts1.NTCSTS_FAILD  SampleTime=inf
  SetNtcSts : Subsystem  RequirementInfo="{'linktype_rmi_doors' '0000babb (/E-STEER Core/SubSystem Specifications/Application Functions/SF053A Handwheel Angle Vehicle Center Trim)' '#SF053A_114' 'true' 'REQ:  SF053A_114' '' } %GIDa_341a4a87_393c_4639_946d_70c5ebaeba98"  mask(SetNTC){}
      mask help: SetNTC library block
  Subtract1 : Sum  RequirementInfo="{'linktype_rmi_doors' '0000babb (/E-STEER Core/SubSystem Specifications/Application Functions/SF053A Handwheel Angle Vehicle Center Trim)' '#SF053A_28' 'true' 'REQ:  SF053A_28' '' } %GIDa_420362e7_c076_4984_bc91_ada16fee1bca"  Inputs=+-
  HwAgVehTrimOffs : Outport  RequirementInfo="{'linktype_rmi_doors' '0000babb (/E-STEER Core/SubSystem Specifications/Application Functions/SF053A Handwheel Angle Vehicle Center Trim)' '#SF053A_28' 'true' 'REQ:  SF053A_28' '' } %GIDa_9911d2e9_4107_4e64_a092_53f256c31f40"
  HwAgTrimPrfmd : Outport  Port=2
  wires:
  Constant3/1 -> SetNtcSts/1(NtcNr)
  HwAg/1 -> Subtract1/1
  HwAgTrimData_Read/1 -> Subtract1/2
  Subtract1/1 -> LimStat_f1/1
  LimStat_f1/1 -> HwAgVehTrimOffs/1
  HwAgTrimData_Read/2 -> If/1, HwAgTrimPrfmd/1
  NtcSts1/1 -> SetNtcSts/3(NtcSts)
  Constant9/1 -> SetNtcSts/4(DebStep)
  Calibration1/1 -> SetNtcSts/2(NtcStInfo)
  If/1 -> SetNtcSts/Action

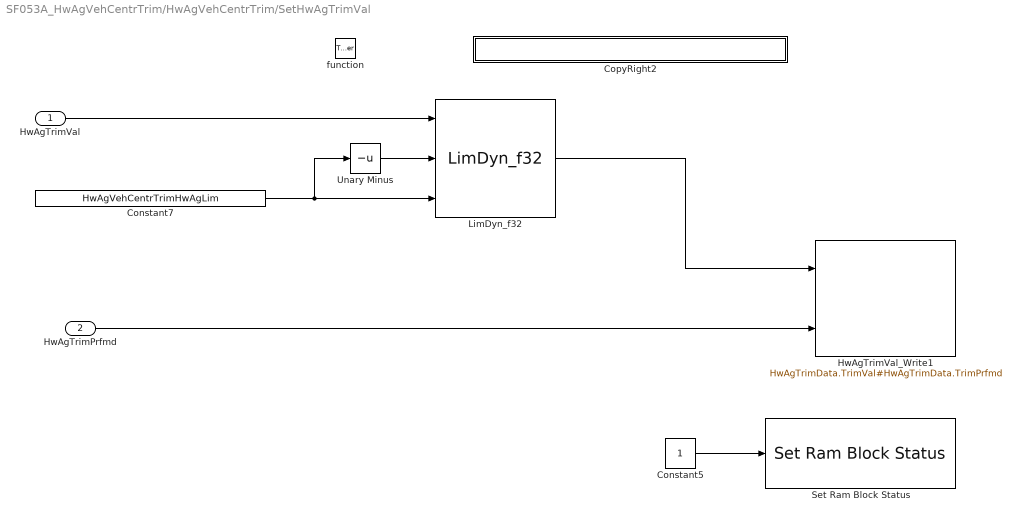
== system SF053A_HwAgVehCentrTrim/HwAgVehCentrTrim/SetHwAgTrimVal ==
  HwAgTrimVal : Inport  RequirementInfo="{'linktype_rmi_doors' '0000babb (/E-STEER Core/SubSystem Specifications/Application Functions/SF053A Handwheel Angle Vehicle Center Trim)' '#SF053A_60' 'true' 'REQ:  SF053A_60' '' } %GIDa_e051215a_d062_47c0_9b78_3ab38dfc1bf9"
  HwAgTrimPrfmd : Inport  RequirementInfo="{'linktype_rmi_doors' '0000babb (/E-STEER Core/SubSystem Specifications/Application Functions/SF053A Handwheel Angle Vehicle Center Trim)' '#SF053A_93' 'true' 'REQ:  SF053A_93' '' } %GIDa_3c6c8a3a_d1a8_49c9_bc68_cf0d7984ee7f"  Port=2
  function : TriggerPort  TriggerType=function-call
  Constant5 : Constant  RequirementInfo="{'linktype_rmi_doors' '0000babb (/E-STEER Core/SubSystem Specifications/Application Functions/SF053A Handwheel Angle Vehicle Center Trim)' '#SF053A_93' 'true' 'REQ:  SF053A_93' '' } %GIDa_d42d9a45_5de1_42b5_aa07_79a88cd15fcd"  OutDataTypeStr=uint8
  Constant7 : Constant  RequirementInfo="{'linktype_rmi_doors' '0000babb (/E-STEER Core/SubSystem Specifications/Application Functions/SF053A Handwheel Angle Vehicle Center Trim)' '#SF053A_60' 'true' 'REQ:  SF053A_60' '' } %GIDa_e92a6ffe_c0aa_4d9b_b6fd_773b5a6280be"  Value=HwAgVehCentrTrimHwAgLim
  CopyRight2 : Subsystem  Description=|  mask(Copyright Information){none=on}
      | Copyright info block.                                               
      |                                                                     
      | Place copyright information at the top of every subsystem in design.
      mask prompts: none "No parameters"
      mask help: Place copyright information at the top of every subsystem in design.
      mask Display:
      | NxtrConf = 'Nexteer Confidential';
      | 
      | sys = bdroot; %handle for the current model ("system")
      | first = get_param(sys,'Created');
      | if(isempty(first))
      |     first = datestr(now,'yyyy');
      | else
      |     first = first(end-3:end);  %year is last four digits
      | end
      | 
      | last = get_param(sys,'LastModifiedDate');
      | if isempty(last)
      |     last = datestr(now,'yyyy');
      | else
      |     last = last(end-3:end);
      | end
      | 
      | if strcmp(first,last)
      |     fprintf('%s -- Copyright %s Nexteer',NxtrConf,first)
      | else
      |     fprintf('%s -- %s%s- %s Nexteer',NxtrConf,char(169),first,last)
      | end
  HwAgTrimVal_Write1 : DataStoreWrite  RequirementInfo="{'linktype_rmi_doors' '0000babb (/E-STEER Core/SubSystem Specifications/Application Functions/SF053A Handwheel Angle Vehicle Center Trim)' '#SF053A_60' 'true' 'REQ:  SF053A_60' '' ; 'linktype_rmi_doors' '0000babb (/E-STEER Core/SubSystem Specifications/Application Functions/SF053A Handwheel Angle Vehicle Center Trim)' '#SF053A_93' 'true' 'REQ:  SF053A_93' '' } %GIDa_c923dece_ba00_4c67_b8f1_2be5261238f7"  DataStoreName=HwAgTrimData  DataStoreElements=HwAgTrimData.TrimVal#HwAgTrimData.TrimPrfmd
  LimDyn_f32 : NxtrLim/LimDyn_f32  RequirementInfo="{'linktype_rmi_doors' '0000babb (/E-STEER Core/SubSystem Specifications/Application Functions/SF053A Handwheel Angle Vehicle Center Trim)' '#SF053A_60' 'true' 'REQ:  SF053A_60' '' } %GIDa_dd8ed54d_56f2_408c_9e89_60b4513da407"
  Set Ram Block Status : NxtrNvM/Set Ram Block Status  RequirementInfo="{'linktype_rmi_doors' '0000babb (/E-STEER Core/SubSystem Specifications/Application Functions/SF053A Handwheel Angle Vehicle Center Trim)' '#SF053A_93' 'true' 'REQ:  SF053A_93' '' } %GIDa_81bd1878_388e_4dd1_b589_5dbde81e0a58"  FuncName=Set Ram Block Status  NvMBlockName=HwAgTrimData  VoidFuncRtn=on  BlockChanged_DSN=NvMSRBS_BlockChanged  Return_DSN=NvMSRBS_Return
      settings: AttributesFormatString=%<FuncName>
  Unary Minus : UnaryMinus  RequirementInfo="{'linktype_rmi_doors' '0000babb (/E-STEER Core/SubSystem Specifications/Application Functions/SF053A Handwheel Angle Vehicle Center Trim)' '#SF053A_60' 'true' 'REQ:  SF053A_60' '' } %GIDa_ed7c7388_44d2_4716_9cc9_1d5d6dcead67"
  wires:
  HwAgTrimVal/1 -> LimDyn_f32/1
  Constant7/1 -> Unary Minus/1, LimDyn_f32/3
  Unary Minus/1 -> LimDyn_f32/2
  LimDyn_f32/1 -> HwAgTrimVal_Write1/1
  Constant5/1 -> Set Ram Block Status/1
  HwAgTrimPrfmd/1 -> HwAgTrimVal_Write1/2

== stateflow chart SF053A_HwAgVehCentrTrim/HwAgVehCentrTrim/UpdHwAgTrimVal/SetNtcSts1/SetNtcSts/ISO Fault Debounce Design ==
  note: NTCSTS_PASSD           (0)
      | NTCSTS_FAILD             (1)
      | NTCSTS_PREPASSD   (2)
      | NTCSTS_PREFAILD     (3)
      |
      | SIGQLFR_NORES        (0)
      | SIGQLFR_PASSD         (1)
      | SIGQLFR_FAILD           (2)
  note: Pass Loop
  note: Fail Loop
  note: 
  (default) -> (junction 89)
  (junction 89) -> (junction 95) [order 1] : [NtcSts ==3]
  (junction 89) -> (junction 93) [order 2] : [NtcSts ==2]
  (junction 89) -> (junction 141) [order 3] : [NtcSts ==1]
      | { ErrAcc = 32767;
      | Qualifier =2;
      |  }
  (junction 89) -> (junction 141) [order 4] : [NtcSts ==0]
      | { ErrAcc = -32768;
      | Qualifier=1;
      | }
  (junction 95) -> (junction 103) [order 2]
  (junction 95) -> (junction 111) [order 1] : [ErrAcc <=0]
      | {ErrAcc = DebStep;}
  (junction 93) -> (junction 123) [order 2] : {
      | ErrAcc = ErrAcc - DebStep;
      | }
  (junction 93) -> (junction 123) [order 1] : [(ErrAcc - DebStep) <= -32768]
      | { ErrAcc = -32768;
      | Qualifier=1;
      | }
  (junction 103) -> (junction 111) [order 1] : [(ErrAcc + DebStep) <32767]
      | {ErrAcc = ErrAcc + DebStep;}
  (junction 103) -> (junction 111) [order 2] : {ErrAcc = 32767;
      | Qualifier =2;}
  (junction 123) -> (junction 141)
  (junction 111) -> (junction 141)
  (junction 141) -> (junction 159) [order 2] : {ErrAcc = 0;
      | Qualifier =0;
      | }
  (junction 141) -> (junction 159) [order 1] : [SvcClr ==0]
  data: NtcSts input Enum: NtcSts1; Qualifier output uint8; DebStep input uint16; ErrAcc local single; SvcClr input

== stateflow chart SF053A_HwAgVehCentrTrim/HwAgVehCentrTrim/UpdHwAgTrimVal/SetNtcSts/SetNtcSts/ISO Fault Debounce Design ==
  note: NTCSTS_PASSD           (0)
      | NTCSTS_FAILD             (1)
      | NTCSTS_PREPASSD   (2)
      | NTCSTS_PREFAILD     (3)
      |
      | SIGQLFR_NORES        (0)
      | SIGQLFR_PASSD         (1)
      | SIGQLFR_FAILD           (2)
  note: Pass Loop
  note: Fail Loop
  note: 
  (default) -> (junction 89)
  (junction 89) -> (junction 95) [order 1] : [NtcSts ==3]
  (junction 89) -> (junction 93) [order 2] : [NtcSts ==2]
  (junction 89) -> (junction 141) [order 3] : [NtcSts ==1]
      | { ErrAcc = 32767;
      | Qualifier =2;
      |  }
  (junction 89) -> (junction 141) [order 4] : [NtcSts ==0]
      | { ErrAcc = -32768;
      | Qualifier=1;
      | }
  (junction 95) -> (junction 103) [order 2]
  (junction 95) -> (junction 111) [order 1] : [ErrAcc <=0]
      | {ErrAcc = DebStep;}
  (junction 93) -> (junction 123) [order 2] : {
      | ErrAcc = ErrAcc - DebStep;
      | }
  (junction 93) -> (junction 123) [order 1] : [(ErrAcc - DebStep) <= -32768]
      | { ErrAcc = -32768;
      | Qualifier=1;
      | }
  (junction 103) -> (junction 111) [order 1] : [(ErrAcc + DebStep) <32767]
      | {ErrAcc = ErrAcc + DebStep;}
  (junction 103) -> (junction 111) [order 2] : {ErrAcc = 32767;
      | Qualifier =2;}
  (junction 123) -> (junction 141)
  (junction 111) -> (junction 141)
  (junction 141) -> (junction 159) [order 2] : {ErrAcc = 0;
      | Qualifier =0;
      | }
  (junction 141) -> (junction 159) [order 1] : [SvcClr ==0]
  data: NtcSts input Enum: NtcSts1; Qualifier output uint8; DebStep input uint16; ErrAcc local single; SvcClr input

== stateflow chart SF053A_HwAgVehCentrTrim/HwAgVehCentrTrim/HwAgVehCentrTrimPer1/SetNtcSts/SetNtcSts/ISO Fault Debounce Design ==
  note: NTCSTS_PASSD           (0)
      | NTCSTS_FAILD             (1)
      | NTCSTS_PREPASSD   (2)
      | NTCSTS_PREFAILD     (3)
      |
      | SIGQLFR_NORES        (0)
      | SIGQLFR_PASSD         (1)
      | SIGQLFR_FAILD           (2)
  note: Pass Loop
  note: Fail Loop
  note: 
  (default) -> (junction 89)
  (junction 89) -> (junction 95) [order 1] : [NtcSts ==3]
  (junction 89) -> (junction 93) [order 2] : [NtcSts ==2]
  (junction 89) -> (junction 141) [order 3] : [NtcSts ==1]
      | { ErrAcc = 32767;
      | Qualifier =2;
      |  }
  (junction 89) -> (junction 141) [order 4] : [NtcSts ==0]
      | { ErrAcc = -32768;
      | Qualifier=1;
      | }
  (junction 95) -> (junction 103) [order 2]
  (junction 95) -> (junction 111) [order 1] : [ErrAcc <=0]
      | {ErrAcc = DebStep;}
  (junction 93) -> (junction 123) [order 2] : {
      | ErrAcc = ErrAcc - DebStep;
      | }
  (junction 93) -> (junction 123) [order 1] : [(ErrAcc - DebStep) <= -32768]
      | { ErrAcc = -32768;
      | Qualifier=1;
      | }
  (junction 103) -> (junction 111) [order 1] : [(ErrAcc + DebStep) <32767]
      | {ErrAcc = ErrAcc + DebStep;}
  (junction 103) -> (junction 111) [order 2] : {ErrAcc = 32767;
      | Qualifier =2;}
  (junction 123) -> (junction 141)
  (junction 111) -> (junction 141)
  (junction 141) -> (junction 159) [order 2] : {ErrAcc = 0;
      | Qualifier =0;
      | }
  (junction 141) -> (junction 159) [order 1] : [SvcClr ==0]
  data: NtcSts input Enum: NtcSts1; Qualifier output uint8; DebStep input uint16; ErrAcc local single; SvcClr input

== stateflow chart SF053A_HwAgVehCentrTrim/HwAgVehCentrTrim/ClrHwAgTrimVal/SetNtcSts/ISO Fault Debounce Design ==
  note: NTCSTS_PASSD           (0)
      | NTCSTS_FAILD             (1)
      | NTCSTS_PREPASSD   (2)
      | NTCSTS_PREFAILD     (3)
      |
      | SIGQLFR_NORES        (0)
      | SIGQLFR_PASSD         (1)
      | SIGQLFR_FAILD           (2)
  note: Pass Loop
  note: Fail Loop
  note: 
  (default) -> (junction 89)
  (junction 89) -> (junction 95) [order 1] : [NtcSts ==3]
  (junction 89) -> (junction 93) [order 2] : [NtcSts ==2]
  (junction 89) -> (junction 141) [order 3] : [NtcSts ==1]
      | { ErrAcc = 32767;
      | Qualifier =2;
      |  }
  (junction 89) -> (junction 141) [order 4] : [NtcSts ==0]
      | { ErrAcc = -32768;
      | Qualifier=1;
      | }
  (junction 95) -> (junction 103) [order 2]
  (junction 95) -> (junction 111) [order 1] : [ErrAcc <=0]
      | {ErrAcc = DebStep;}
  (junction 93) -> (junction 123) [order 2] : {
      | ErrAcc = ErrAcc - DebStep;
      | }
  (junction 93) -> (junction 123) [order 1] : [(ErrAcc - DebStep) <= -32768]
      | { ErrAcc = -32768;
      | Qualifier=1;
      | }
  (junction 103) -> (junction 111) [order 1] : [(ErrAcc + DebStep) <32767]
      | {ErrAcc = ErrAcc + DebStep;}
  (junction 103) -> (junction 111) [order 2] : {ErrAcc = 32767;
      | Qualifier =2;}
  (junction 123) -> (junction 141)
  (junction 111) -> (junction 141)
  (junction 141) -> (junction 159) [order 2] : {ErrAcc = 0;
      | Qualifier =0;
      | }
  (junction 141) -> (junction 159) [order 1] : [SvcClr ==0]
  data: NtcSts input Enum: NtcSts1; Qualifier output uint8; DebStep input uint16; ErrAcc local single; SvcClr input

== stateflow chart SF053A_HwAgVehCentrTrim/HwAgVehCentrTrim/HwAgVehCentrTrimInit1/SetNtcSts/SetNtcSts/ISO Fault Debounce Design ==
  note: NTCSTS_PASSD           (0)
      | NTCSTS_FAILD             (1)
      | NTCSTS_PREPASSD   (2)
      | NTCSTS_PREFAILD     (3)
      |
      | SIGQLFR_NORES        (0)
      | SIGQLFR_PASSD         (1)
      | SIGQLFR_FAILD           (2)
  note: Pass Loop
  note: Fail Loop
  note: 
  (default) -> (junction 89)
  (junction 89) -> (junction 95) [order 1] : [NtcSts ==3]
  (junction 89) -> (junction 93) [order 2] : [NtcSts ==2]
  (junction 89) -> (junction 141) [order 3] : [NtcSts ==1]
      | { ErrAcc = 32767;
      | Qualifier =2;
      |  }
  (junction 89) -> (junction 141) [order 4] : [NtcSts ==0]
      | { ErrAcc = -32768;
      | Qualifier=1;
      | }
  (junction 95) -> (junction 103) [order 2]
  (junction 95) -> (junction 111) [order 1] : [ErrAcc <=0]
      | {ErrAcc = DebStep;}
  (junction 93) -> (junction 123) [order 2] : {
      | ErrAcc = ErrAcc - DebStep;
      | }
  (junction 93) -> (junction 123) [order 1] : [(ErrAcc - DebStep) <= -32768]
      | { ErrAcc = -32768;
      | Qualifier=1;
      | }
  (junction 103) -> (junction 111) [order 1] : [(ErrAcc + DebStep) <32767]
      | {ErrAcc = ErrAcc + DebStep;}
  (junction 103) -> (junction 111) [order 2] : {ErrAcc = 32767;
      | Qualifier =2;}
  (junction 123) -> (junction 141)
  (junction 111) -> (junction 141)
  (junction 141) -> (junction 159) [order 2] : {ErrAcc = 0;
      | Qualifier =0;
      | }
  (junction 141) -> (junction 159) [order 1] : [SvcClr ==0]
  data: NtcSts input Enum: NtcSts1; Qualifier output uint8; DebStep input uint16; ErrAcc local single; SvcClr input
